simulink model "UAV_sync_known_sim"  (R2018b)
settings: Solver=ode23tb  StartTime=0.0  StopTime=35
values from neighbouring files (symbols this model uses):
  C_rho = 1.225    [SC42120_UAV_Preconditions.m]
  D0 = [M0 0 0 0 0 0 ... (first row only)    [SC42120_UAV_Preconditions.m]
  Derivative_gain_phi = 50    [SC42120_UAV_Preconditions.m]
  Derivative_gain_psi = 50    [SC42120_UAV_Preconditions.m]
  Derivative_gain_theta = 50    [SC42120_UAV_Preconditions.m]
  Derivative_gain_x = 50    [SC42120_UAV_Preconditions.m]
  Derivative_gain_y = 50    [SC42120_UAV_Preconditions.m]
  Derivative_gain_z = 50    [SC42120_UAV_Preconditions.m]
  G = 9.80665    [SC42120_UAV_Preconditions.m]
  g0 = [0;0;-M0*G;0;0;0]    [SC42120_UAV_Preconditions.m]
  I0 = [0.02 0 -0.01 ... (first row only)    [SC42120_UAV_Preconditions.m]
  I1 = [0.1 0 -0.01;0 0.05 0;-0.01 0 0.1]    [UAV_sync_known.m]    (also in UAV_sync_unknown.m; UAV_sync_unknown_Node1.m)
  InitWind = [0;0;0]    [SC42120_UAV_Preconditions.m]
  M0 = 10    [SC42120_UAV_Preconditions.m]
  M1 = 20    [UAV_sync_known.m]    (also in UAV_sync_unknown.m; UAV_sync_unknown_Node1.m)
  Proportional_phi = 50    [SC42120_UAV_Preconditions.m]
  Proportional_psi = 50    [SC42120_UAV_Preconditions.m]
  Proportional_theta = 50    [SC42120_UAV_Preconditions.m]
  Proportional_x = 50    [SC42120_UAV_Preconditions.m]
  Proportional_y = 50    [SC42120_UAV_Preconditions.m]
  Proportional_z = 50    [SC42120_UAV_Preconditions.m]
undefined symbols (not defined in the file or in its folder): Aero, APlane, Bxl, C, Ctr, deg, DiscIntNeverNeededParam, F, Guid, Init, Light, MIL, Path, rad, s, Trim, Utility
libraries: aerolibconvert2 x37, simulink x15, dspsigops x7, shared6dof x6, aerolibasang x4, simulink_extras x3, aerolibadyn x1, aerolibtransform2 x1, aerolibwind2 x1
(part 1 of 6)
settings Model: Creator=Muhammad Ridho Rosa  LastModifiedBy=Jesse
settings SolverCC: ZeroCrossAlgorithm=Adaptive
settings SFSimCC: SimUseLocalCustomCode=off
settings RTWCC: RTWUseLocalCustomCode=off
settings CodeAppCC: StateflowObjectComments=on

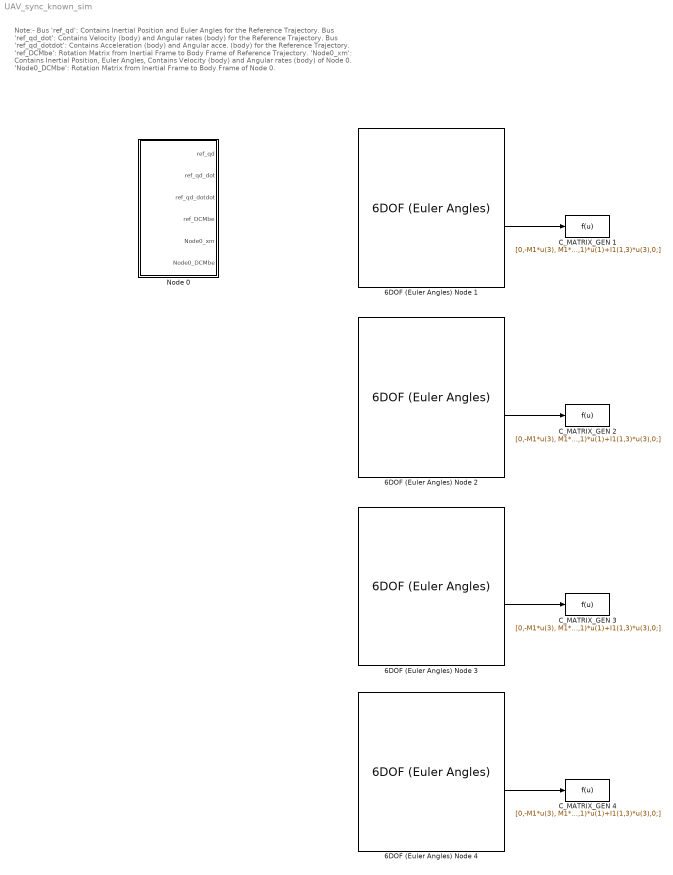
== system UAV_sync_known_sim ==
  note: Note:-
      | Bus 'ref_qd': Contains Inertial Position and Euler Angles for the Reference Trajectory.
      | Bus 'ref_qd_dot': Contains Velocity (body) and Angular rates (body) for the Reference Trajectory.
      | Bus 'ref_qd_dotdot': Contains Acceleration (body) and Angular acce. (body) for the Reference Trajectory.
      | 'ref_DCMbe': Rotation Matrix from Inertial Frame to Body Frame of Reference Trajectory.
      | 'Node0_xm': Contains Inertial Position, Euler Angles, Contains Velocity (body) and Angular rates (body) of Node 0.
      | 'Node0_DCMbe': Rotation Matrix from Inertial Frame to Body Frame of Node 0.
  6DOF (Euler Angles) Node 1 : shared6dof/6DOF (Euler Angles)  units=Metric (MKS)  mtype=Fixed  rep=Euler Angles  xme_0=init_pos1  Vm_0=init_vel1  eul_0=init_eul1  pm_0=init_ang1  mass_0=M1  mass_e=0.5  mass_f=2.0  inertia=I1  inertia_e=eye(3)  inertia_f=2*eye(3)  k_quat=1.0  vre_flag=on  abi_flag=on  aMode=0  xme_statename=''  Vm_statename=''  eul_statename=''  quat_statename=''  pm_statename=''  mass_statename=''
      settings: SourceProductBaseCode=AE
  6DOF (Euler Angles) Node 2 : shared6dof/6DOF (Euler Angles)  units=Metric (MKS)  mtype=Fixed  rep=Euler Angles  xme_0=init_pos2  Vm_0=init_vel2  eul_0=init_eul2  pm_0=init_ang2  mass_0=M2  mass_e=0.5  mass_f=2.0  inertia=I2  inertia_e=eye(3)  inertia_f=2*eye(3)  k_quat=1.0  vre_flag=on  abi_flag=on  aMode=0  xme_statename=''  Vm_statename=''  eul_statename=''  quat_statename=''  pm_statename=''  mass_statename=''
      settings: SourceProductBaseCode=AE
  6DOF (Euler Angles) Node 3 : shared6dof/6DOF (Euler Angles)  units=Metric (MKS)  mtype=Fixed  rep=Euler Angles  xme_0=init_pos3  Vm_0=init_vel3  eul_0=init_eul3  pm_0=init_ang3  mass_0=M3  mass_e=0.5  mass_f=2.0  inertia=I3  inertia_e=eye(3)  inertia_f=2*eye(3)  k_quat=1.0  vre_flag=on  abi_flag=on  aMode=0  xme_statename=''  Vm_statename=''  eul_statename=''  quat_statename=''  pm_statename=''  mass_statename=''
      settings: SourceProductBaseCode=AE
  6DOF (Euler Angles) Node 4 : shared6dof/6DOF (Euler Angles)  units=Metric (MKS)  mtype=Fixed  rep=Euler Angles  xme_0=init_pos4  Vm_0=init_vel4  eul_0=init_eul4  pm_0=init_ang4  mass_0=M4  mass_e=0.5  mass_f=2.0  inertia=I4  inertia_e=eye(3)  inertia_f=2*eye(3)  k_quat=1.0  vre_flag=on  abi_flag=on  aMode=0  xme_statename=''  Vm_statename=''  eul_statename=''  quat_statename=''  pm_statename=''  mass_statename=''
      settings: SourceProductBaseCode=AE
  C_MATRIX_GEN {1..4} (4 alike) : Fcn  Expr=[0,-M1*u(3), M1*u(2), 0,0,0; M1*u(3),0,-M1*u(1),0,0,0;-M1*u(2),M1*u(1),0,0,0,0;0,0,0,0,I1(3,3)*u(3)-I1(1,3)*u(1),-I1(2,2)*u(2);0,0,0,-I1(3,3)*u(3)+I1(1,3)*u(1),0,I1(1,1)*u(1)-I1(1,3)*u(3);0,0,0,I1(2,2)*u(2),-I1(1,1)*u(1)+I1(1,3)*u(3),0;]
  Node 0 : Subsystem
  wires:
  6DOF (Euler Angles) Node 1/6 -> C_MATRIX_GEN 1/1
  6DOF (Euler Angles) Node 2/6 -> C_MATRIX_GEN 2/1
  6DOF (Euler Angles) Node 3/6 -> C_MATRIX_GEN 3/1
  6DOF (Euler Angles) Node 4/6 -> C_MATRIX_GEN 4/1

== system UAV_sync_known_sim/Node 0 ==
  Bus Creator : BusCreator  Inputs=2
  Bus Creator1 : BusCreator  Inputs=2
  Bus Creator2 : BusCreator  Inputs=2
  Bus Creator3 : BusCreator  Inputs=4
  Bus Selector : BusSelector  OutputSignals=PlantData.Position (inertial),PlantData.Euler angles (rad),PlantData.Velocity (body),PlantData.Angular rates (body) (rad/s),PlantData.Accelerations (body/body),PlantData.Angular accelerations (body/body),PlantData.From inertial to body matrix
  Bus Selector1 : BusSelector  OutputSignals=Position (inertial),Euler angles (rad),Velocity (body),Angular rates (body),MatrixTransformation(Inertial-Body)
  Node 0 : Subsystem
  VF Approach : Subsystem
  ref_qd : Outport
  ref_qd_dot : Outport  Port=2
  ref_qd_dotdot : Outport  Port=3
  ref_DCMbe : Outport  Port=4
  Node0_xm : Outport  Port=5
  Node0_DCMbe : Outport  Port=6
  wires:
  VF Approach/1(VF_System_Parameters) -> Node 0/1(VF_System_Parameters)
  VF Approach/2(PlantData) -> Bus Selector/1
  Bus Selector/1 -> Bus Creator/1  "<Position (inertial)>"
  Bus Selector/2 -> Bus Creator/2  "<Euler angles (rad)>"
  Bus Creator/1 -> ref_qd/1
  Bus Selector/4 -> Bus Creator1/2  "<Angular rates (body) (rad/s)>"
  Bus Selector/3 -> Bus Creator1/1  "<Velocity (body)>"
  Bus Creator1/1 -> ref_qd_dot/1
  Bus Selector/6 -> Bus Creator2/2  "<Angular accelerations (body/body)>"
  Bus Selector/5 -> Bus Creator2/1  "<Accelerations (body/body)>"
  Bus Creator2/1 -> ref_qd_dotdot/1
  Bus Selector/7 -> ref_DCMbe/1  "<From inertial to body matrix>"
  Node 0/1(Node0_Data) -> Bus Selector1/1
  Bus Selector1/1 -> Bus Creator3/1  "<Position (inertial)>"
  Bus Selector1/3 -> Bus Creator3/3  "<Velocity (body)>"
  Bus Selector1/4 -> Bus Creator3/4  "<Angular rates (body)>"
  Bus Creator3/1 -> Node0_xm/1
  Bus Selector1/5 -> Node0_DCMbe/1  "<MatrixTransformation(Inertial-Body)>"
  Bus Selector1/2 -> Bus Creator3/2  "<Euler angles (rad)>"

== system UAV_sync_known_sim/Node 0/Node 0 ==
  note: Inverse Dynamics
  VF_System_Parameters : Inport
  6DOF (Euler Angles) : shared6dof/6DOF (Euler Angles)  units=Metric (MKS)  mtype=Fixed  rep=Euler Angles  xme_0=init_pos0  Vm_0=init_vel0  eul_0=init_eul0  pm_0=init_ang0  mass_0=M0  mass_e=0.5  mass_f=2.0  inertia=I0  inertia_e=eye(3)  inertia_f=2*eye(3)  k_quat=1.0  vre_flag=on  abi_flag=off  aMode=aMode  xme_statename=''  Vm_statename=''  eul_statename=''  quat_statename=''  pm_statename=''  mass_statename=''
      settings: SourceProductBaseCode=AE
  ALL_DATA2 : Goto  Commented=on  GotoTag=DERIVED_DATA
  Add : Sum
  Bus Creator : BusCreator  Inputs=10
  Constant8 : Constant  Value=M0*G
  Demux5 : Demux  Outputs=6
  Derived Data : Subsystem
  Gain : Gain  Gain=[1 1 -1]
  Inverse Dynamics Control : Subsystem
  Mux8 : Mux  Inputs=3
  Mux9 : Mux  Inputs=3
  Product : Product  Multiplication=Matrix(*)
  Subsystem : Subsystem
  Wind : Subsystem
  tau : Sum  Inputs=+++
  Node0_Data : Outport
  wires:
  Gain/1 -> Product/2, Bus Creator/3  "xyh"
  6DOF (Euler Angles)/1 -> Bus Creator/1  "Velocity (inertial)"
  Mux8/1 -> 6DOF (Euler Angles)/1
  6DOF (Euler Angles)/3 -> Bus Creator/4  "Euler angles (rad)"
  Bus Creator/1 -> [AIRCRAFT_DATA]
  6DOF (Euler Angles)/6 -> Bus Creator/7  "Angular rates (body)"
  6DOF (Euler Angles)/8 -> Bus Creator/9  "Acceleration (Body)"
  Mux9/1 -> 6DOF (Euler Angles)/2
  6DOF (Euler Angles)/7 -> Bus Creator/8  "Angular accelerations (body)"
  6DOF (Euler Angles)/5 -> Bus Creator/6  "Velocity (body)"
  6DOF (Euler Angles)/2 -> Gain/1, Bus Creator/2  "Position (inertial)"
  6DOF (Euler Angles)/4 -> Product/1, Bus Creator/5  "MatrixTransformation(Inertial-Body)"
  tau/1 -> Demux5/1
  Demux5/2 -> Mux8/2
  Demux5/4 -> Mux9/1
  Demux5/5 -> Mux9/2
  Demux5/6 -> Mux9/3
  [WIND_DATA] -> Derived Data/1(In1)
  [AIRCRAFT_DATA] -> Derived Data/2(In2)
  Derived Data/1(Derived_Condition) -> ALL_DATA2/1
  [AIRCRAFT_DATA] -> Wind/1(In1)
  Wind/1(Out1) -> [WIND_DATA]
  Inverse Dynamics Control/1(D_qddot) -> tau/1
  Inverse Dynamics Control/2(C_qdot) -> tau/2
  Inverse Dynamics Control/3(g(q)) -> tau/3
  Constant8/1 -> Add/2
  Demux5/3 -> Add/1
  Add/1 -> Mux8/3
  Demux5/1 -> Mux8/1
  [AIRCRAFT_DATA] -> Inverse Dynamics Control/2(Aircraft Data), Node0_Data/1
  VF_System_Parameters/1 -> Subsystem/1(VF_System_Parameters)
  Subsystem/1(References) -> Inverse Dynamics Control/1(References)
  Product/1 -> Bus Creator/10  "xyh_body"

== system UAV_sync_known_sim/Node 0/VF Approach ==
  note: Created by: Stefano Farì
      | Last edit: Mar 2018
  note: Fixed-wing UAV Simulator
  note: Ground Hit
  note: Wind
  note: To workspace
  note: MAIN
  AUTOPILOT : Subsystem
  BIXLER DYNAMICS : Subsystem
  Bus Selector3 : BusSelector  OutputSignals=PlantData.xyh_body,PlantData.Euler angles (rad),PlantData.Velocity (body),PlantData.Angular rates (body) (rad/s),PlantData.Accelerations (body/body),PlantData.Angular accelerations (body/body)
  ENVIRONMENT : Subsystem
  GROUND HIT : Subsystem
  MANUAL INPUTS : Subsystem
  Mux : Mux  Inputs=6
  PATH FOLLOWING : Subsystem
  PATH MANAGER : Subsystem
  TO WORKSPACE : Subsystem
  VF_System_Parameters : Outport
  PlantData : Outport  Port=2
  wires:
  MANUAL INPUTS/2(EnvData.) -> BIXLER DYNAMICS/2(EnvData)
  [PlantData] -> PATH MANAGER/1(PlantData)
  MANUAL INPUTS/4(VF.) -> BIXLER DYNAMICS/4(VF)
  [VF] -> TO WORKSPACE/4(VF)
  MANUAL INPUTS/3(GuidData.) -> BIXLER DYNAMICS/3(GuidData)
  [EnvData] -> PATH MANAGER/3(EnvData)
  [PlantData] -> PlantData/1, Bus Selector3/1
  BIXLER DYNAMICS/4(GuidData.) -> [GuidData]
  MANUAL INPUTS/1(CtrBus.) -> BIXLER DYNAMICS/1(ControlActions)
  AUTOPILOT/3(VF.) -> MANUAL INPUTS/3(VF)
  PATH MANAGER/2(DerCond.) -> PATH FOLLOWING/2(DerCond)
  PATH FOLLOWING/1("PlantData. ") -> AUTOPILOT/1(PlantData)
  AUTOPILOT/4(GuidData.) -> MANUAL INPUTS/4(GuidData)
  [GuidData] -> TO WORKSPACE/5(GuidData)
  [DerCond] -> TO WORKSPACE/2(DerCond)
  PATH FOLLOWING/5(GuidData.) -> AUTOPILOT/5(GuidData)
  BIXLER DYNAMICS/5(VF.) -> [VF]
  PATH FOLLOWING/2("DerCond. ") -> AUTOPILOT/2(DerCond)
  BIXLER DYNAMICS/1(PlantData.) -> [PlantData]
  [PlantData] -> GROUND HIT/1(PlantData)
  [PlantData] -> ENVIRONMENT/1(PlantData)
  BIXLER DYNAMICS/3(ControlBus.) -> [ControlBus]
  AUTOPILOT/2(EnvData.) -> MANUAL INPUTS/2(EnvData)
  PATH MANAGER/1(Plantdata.) -> PATH FOLLOWING/1(PlantData)
  PATH MANAGER/4(GuidData.) -> PATH FOLLOWING/4(GuidData)
  ENVIRONMENT/1(EnvData) -> [EnvData]
  PATH FOLLOWING/4(VF.) -> AUTOPILOT/4(VF)
  Bus Selector3/4 -> Mux/4  "<Angular rates (body) (rad/s)>"
  PATH MANAGER/3(EnvData.) -> PATH FOLLOWING/3(EnvData)
  [PlantData] -> TO WORKSPACE/1(PlantData)
  [DerCond] -> PATH MANAGER/2(DerCond)
  BIXLER DYNAMICS/2(DerCond.) -> [DerCond]
  [EnvData] -> TO WORKSPACE/6(EnvData)
  [ControlBus] -> TO WORKSPACE/3(ControlBus)
  AUTOPILOT/1(CtrBus.) -> MANUAL INPUTS/1(CtrBus)
  PATH FOLLOWING/3(EnvData.) -> AUTOPILOT/3(EnvData)
  Mux/1 -> VF_System_Parameters/1
  Bus Selector3/1 -> Mux/1  "<xyh_body>"
  Bus Selector3/2 -> Mux/2  "<Euler angles (rad)>"
  Bus Selector3/3 -> Mux/3  "<Velocity (body)>"
  Bus Selector3/5 -> Mux/5  "<Accelerations (body/body)>"
  Bus Selector3/6 -> Mux/6  "<Angular accelerations (body/body)>"

== system UAV_sync_known_sim/Node 0/Node 0/Derived Data ==
  note: WAE = Wind Angle Error
  In1 : Inport
  In2 : Inport  Port=2
  Bus Creator2 : BusCreator  Inputs=7
  Bus Selector : BusSelector  OutputSignals=WindVelocity(Body)
  Bus Selector5 : BusSelector  OutputSignals=Velocity (body),Velocity (inertial),Euler angles (rad)
  Constant9 : Constant  Value=C_rho
  Dynamic Pressure : aerolibasang/Dynamic Pressure
  "Incidence, Sideslip, & Airspeed" : aerolibasang/Incidence, Sideslip, & Airspeed
      settings: SourceProductName=Aerospace Blockset
  Scope : Scope
  Selector : Selector  InputPortWidth=3  IndexOptions=Index vector (dialog)  Indices=3  OutputSizes=1
  Selector1 : Selector  InputPortWidth=3  IndexOptions=Index vector (dialog)  Indices=2  OutputSizes=1
  Selector3 : Selector  InputPortWidth=3  IndexOptions=Index vector (dialog)  Indices=1  OutputSizes=1
  Sum2 : Sum  Inputs=|-+
  Sum4 : Sum  Inputs=+-|
  Sum5 : Sum  Inputs=+-|
  Trigonometric Function1 : Trigonometry  Operator=atan2
  Derived_Condition : Outport
  wires:
  In2/1 -> Bus Selector5/1
  "Incidence, Sideslip, & Airspeed"/2 -> Sum5/2, Bus Creator2/2  "beta"
  "Incidence, Sideslip, & Airspeed"/1 -> Bus Creator2/1  "alpha"
  Dynamic Pressure/1 -> Bus Creator2/4  "qbar"
  Sum2/1 -> "Incidence, Sideslip, & Airspeed"/1
  Constant9/1 -> Dynamic Pressure/2
  Bus Selector5/2 -> Selector1/1, Selector3/1  "<Velocity (inertial)>"
  Trigonometric Function1/1 -> Sum4/1, Bus Creator2/5  "course_angle"
  Bus Selector5/3 -> Selector/1  "<Euler angles (rad)>"
  Selector/1 -> Sum4/2
  Sum5/1 -> Bus Creator2/7  "WAE"
  "Incidence, Sideslip, & Airspeed"/3 -> Scope/1, Bus Creator2/3  "Va"
  Sum4/1 -> Sum5/1, Bus Creator2/6  "crab_angle"
  Bus Selector5/1 -> Dynamic Pressure/1, Sum2/2  "<Velocity (body)>"
  Bus Creator2/1 -> Derived_Condition/1
  In1/1 -> Bus Selector/1
  Bus Selector/1 -> Sum2/1  "<WindVelocity(Body)>"
  Selector1/1 -> Trigonometric Function1/1
  Selector3/1 -> Trigonometric Function1/2

== system UAV_sync_known_sim/Node 0/Node 0/Inverse Dynamics Control ==
  References : Inport
  Aircraft Data : Inport  Port=2
  Constant8 : Constant  Value=g0
  Inverse Dynamic 1 : Subsystem
  Inverse Dynamic 2 : Subsystem
  D_qddot : Outport
  C_qdot : Outport  Port=2
  g(q) : Outport  Port=3
  wires:
  Inverse Dynamic 1/1(D_qddot) -> D_qddot/1
  References/1 -> Inverse Dynamic 1/1(References)
  Aircraft Data/1 -> Inverse Dynamic 2/1(Aricraft Data), Inverse Dynamic 1/2(Aircraft Data)
  Inverse Dynamic 2/1(C_qdot) -> C_qdot/1
  Constant8/1 -> g(q)/1

== system UAV_sync_known_sim/Node 0/Node 0/Subsystem ==
  VF_System_Parameters : Inport
  Bus Creator1 : BusCreator  Inputs=18
  Demux : Demux  Outputs=18
  References : Outport
  wires:
  VF_System_Parameters/1 -> Demux/1
  Demux/7 -> Bus Creator1/7  "xdot_ref_final"
  Demux/6 -> Bus Creator1/6  "psi_ref_final"
  Demux/9 -> Bus Creator1/9  "hdot_ref_final"
  Demux/18 -> Bus Creator1/18  "psiddot_ref_final"
  Bus Creator1/1 -> References/1
  Demux/1 -> Bus Creator1/1  "x_ref _final"
  Demux/4 -> Bus Creator1/4  "phi_ref_final"
  Demux/5 -> Bus Creator1/5  "theta_ref_final"
  Demux/2 -> Bus Creator1/2  "y_ref_final"
  Demux/3 -> Bus Creator1/3  "h_ref_final"
  Demux/8 -> Bus Creator1/8  "ydot_ref_final"
  Demux/14 -> Bus Creator1/14  "yddot_ref_final"
  Demux/16 -> Bus Creator1/16  "phiddot_ref_final"
  Demux/15 -> Bus Creator1/15  "hddot_ref_final"
  Demux/10 -> Bus Creator1/10  "phidot_ref_final"
  Demux/13 -> Bus Creator1/13  "xddot_ref_final"
  Demux/17 -> Bus Creator1/17  "thetaddot_ref_final"
  Demux/12 -> Bus Creator1/12  "psidot_ref_final"
  Demux/11 -> Bus Creator1/11  "thetadot_ref_final"

== system UAV_sync_known_sim/Node 0/Node 0/Wind ==
  In1 : Inport
  Bus Creator1 : BusCreator  Inputs=1
  Bus Selector4 : BusSelector  OutputSignals=MatrixTransformation(Inertial-Body)
  Constant1 : Constant  Value=InitWind
  Product : Product  Multiplication=Matrix(*)
  Out1 : Outport
  wires:
  Constant1/1 -> Product/2
  In1/1 -> Bus Selector4/1
  Bus Selector4/1 -> Product/1  "<MatrixTransformation(Inertial-Body)>"
  Product/1 -> Bus Creator1/1  "WindVelocity(Body)"
  Bus Creator1/1 -> Out1/1

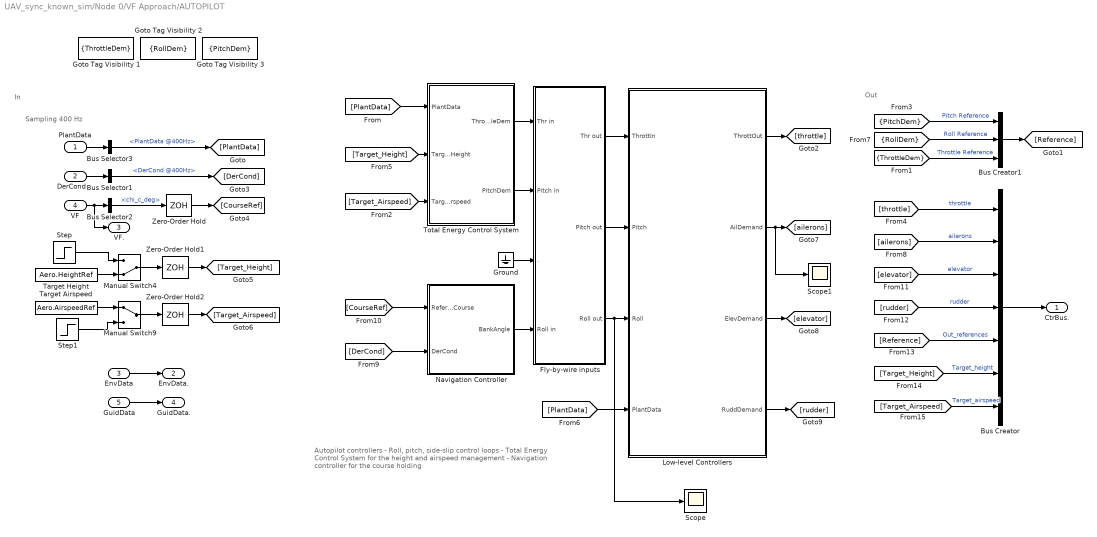
== system UAV_sync_known_sim/Node 0/VF Approach/AUTOPILOT ==
  note: In
  note: Out
  note: Autopilot controllers
      |
      | - Roll, pitch, side-slip control loops
      | - Total Energy Control System for the height and airspeed management
      | - Navigation controller for the course holding
  note: Sampling 400 Hz
  PlantData : Inport
  DerCond : Inport  Port=2
  EnvData : Inport  Port=3
  VF : Inport  Port=4
  GuidData : Inport  Port=5
  Bus Creator : BusCreator  Inputs=7
  Bus Creator1 : BusCreator  Inputs=3
  Bus Selector1 : BusSelector  OutputSignals=DerCond @400Hz
  Bus Selector2 : BusSelector  OutputSignals=chi_c_deg
  Bus Selector3 : BusSelector  OutputSignals=PlantData @400Hz
  Fly-by-wire inputs : Subsystem
  Goto Tag Visibility 1 : GotoTagVisibility  GotoTag=ThrottleDem
  Goto Tag Visibility 2 : GotoTagVisibility  GotoTag=RollDem
  Goto Tag Visibility 3 : GotoTagVisibility  GotoTag=PitchDem
  Ground : Ground
  Low-level Controllers : Subsystem
  Manual Switch4 : ManualSwitch  CurrentSetting=0
  Manual Switch9 : ManualSwitch
  Navigation Controller : Subsystem
  Scope : Scope
  Scope1 : Scope
  Step : Step  Time=10  Before=50  After=80  SampleTime=0
  Step1 : Step  Time=10  Before=15  After=20  SampleTime=0
  Target Airspeed : Constant  Value=Aero.AirspeedRef
  Target Height : Constant  Value=Aero.HeightRef
  Total Energy Control System : Subsystem
  Zero-Order Hold : ZeroOrderHold  SampleTime=1/400
  Zero-Order Hold1 : ZeroOrderHold  SampleTime=1/400
  Zero-Order Hold2 : ZeroOrderHold  SampleTime=1/400
  CtrBus. : Outport
  EnvData. : Outport  Port=2
  VF. : Outport  Port=3
  GuidData. : Outport  Port=4
  wires:
  Bus Creator1/1 -> [Reference]
  PlantData/1 -> Bus Selector3/1
  Low-level Controllers/4(RuddDemand) -> [rudder]
  Low-level Controllers/3(ElevDemand) -> [elevator]
  Low-level Controllers/2(AilDemand) -> Scope1/1, [ailerons]
  Low-level Controllers/1(ThrottOut) -> [throttle]
  [RollDem] -> Bus Creator1/2  "Roll Reference"
  [CourseRef] -> Navigation Controller/1(ReferenceCourse)
  [PlantData] -> Low-level Controllers/4(PlantData)
  Bus Selector1/1 -> [DerCond]  "<DerCond @400Hz>"
  DerCond/1 -> Bus Selector1/1
  [DerCond] -> Navigation Controller/2(DerCond)
  Bus Selector3/1 -> [PlantData]  "<PlantData @400Hz>"
  Manual Switch4/1 -> Zero-Order Hold1/1
  Manual Switch9/1 -> Zero-Order Hold2/1
  Step/1 -> Manual Switch4/1
  Target Height/1 -> Manual Switch4/2
  Target Airspeed/1 -> Manual Switch9/1
  Step1/1 -> Manual Switch9/2
  [PitchDem] -> Bus Creator1/1  "Pitch Reference"
  Zero-Order Hold/1 -> [CourseRef]
  [PlantData] -> Total Energy Control System/1(PlantData)
  EnvData/1 -> EnvData./1
  GuidData/1 -> GuidData./1
  VF/1 -> VF./1, Bus Selector2/1
  Bus Selector2/1 -> Zero-Order Hold/1  "<chi_c_deg>"
  [ThrottleDem] -> Bus Creator1/3  "Throttle Reference"
  Zero-Order Hold1/1 -> [Target_Height]
  Zero-Order Hold2/1 -> [Target_Airspeed]
  Total Energy Control System/1(ThrottleDem) -> Fly-by-wire inputs/1(Thr in)
  Total Energy Control System/2(PitchDem) -> Fly-by-wire inputs/2(Pitch in)
  Navigation Controller/1(BankAngle) -> Fly-by-wire inputs/4(Roll in)
  Fly-by-wire inputs/1(Thr out) -> Low-level Controllers/1(ThrottIn)
  Fly-by-wire inputs/2(Pitch out) -> Low-level Controllers/2(Pitch)
  Ground/1 -> Fly-by-wire inputs/3(.)
  [Target_Height] -> Total Energy Control System/2(Target_Height)
  [Target_Airspeed] -> Total Energy Control System/3(Target_Airspeed)
  [ailerons] -> Bus Creator/2  "ailerons"
  [throttle] -> Bus Creator/1  "throttle"
  [elevator] -> Bus Creator/3  "elevator"
  [rudder] -> Bus Creator/4  "rudder"
  [Reference] -> Bus Creator/5  "Out_references"
  [Target_Height] -> Bus Creator/6  "Target_height"
  [Target_Airspeed] -> Bus Creator/7  "Target_airspeed"
  Bus Creator/1 -> CtrBus./1
  Fly-by-wire inputs/3(Roll out) -> Low-level Controllers/3(Roll), Scope/1

== system UAV_sync_known_sim/Node 0/VF Approach/BIXLER DYNAMICS ==
  note: This sub-block contains the dynamics of the aircraft.
      |
      | - All the states and quantities of interest are contained in the Bus signal PlantData.
      | - The derived conditions such as Airspeed, Angle of Attack, and Side-slip angle, are contained in Bus signal DerCond .
      | - The Bus EnvData contains the wind quantities of interest.
      | - The dynamical model is continuous, but the Buses are sampled to feed the discrete-time control system.
      | - The parameters of this block are contained in parameters/parameters_aero.
  ControlActions : Inport
  EnvData : Inport  Port=2
  GuidData : Inport  Port=3
  VF : Inport  Port=4
  Actuator Dynamics : Subsystem
  Bus Creator1 : BusCreator  Inputs='qbar','alpha','beta','Va','Course','CrabAngle','WAE'
  Bus Selector : BusSelector  OutputSignals=throttle
  Derived Conditions : Subsystem
  RUBBISH BIN : Subsystem
  Sampling : Subsystem
  "Sampling " : Subsystem
  Throttle Dynamics : Subsystem
  Vehicle Airframe : Subsystem
  PlantData. : Outport
  DerCond. : Outport  Port=2
  ControlBus. : Outport  Port=3
  GuidData. : Outport  Port=4
  VF. : Outport  Port=5
  wires:
  Bus Creator1/1 -> "Sampling "/1(Cont.), [DerCond]  "DerCond"
  Bus Selector/1 -> Throttle Dynamics/1(In)  "<throttle>"
  Throttle Dynamics/1(Out) -> Vehicle Airframe/1(Throttle_cmd)  "throttle"
  ControlActions/1 -> ControlBus./1, Bus Selector/1, Actuator Dynamics/1(In)
  Actuator Dynamics/1(Out) -> Vehicle Airframe/2(ControlActions)
  Vehicle Airframe/1(PlantData) -> [PlantData], Sampling/1(Cont.)  "PlantData"
  Sampling/1(Cont.+Disc.) -> PlantData./1
  "Sampling "/1(Cont.+Disc.) -> DerCond./1
  GuidData/1 -> GuidData./1
  VF/1 -> VF./1
  [PlantData] -> Derived Conditions/2(PlantData)
  EnvData/1 -> Derived Conditions/1(EnvData)
  Derived Conditions/1(qbar) -> Bus Creator1/1  "qbar"
  Derived Conditions/2(alpha) -> Bus Creator1/2  "alpha"
  Derived Conditions/4(Va) -> Bus Creator1/4  "Va"
  Derived Conditions/3(beta) -> Bus Creator1/3  "beta"
  Derived Conditions/5(CourseAngle) -> Bus Creator1/5  "Course"
  Derived Conditions/6(CrabAngle) -> Bus Creator1/6  "CrabAngle"
  Derived Conditions/7(WAE) -> Bus Creator1/7  "WAE"
  [DerCond] -> Vehicle Airframe/3(DerCond)

== system UAV_sync_known_sim/Node 0/VF Approach/ENVIRONMENT ==
  note: Wind slowly time varying
  note: Dynamic wind
  note: Constant wind
  PlantData : Inport
  Bus Creator : BusCreator  Inputs=4
  Bus Selector1 : BusSelector  OutputSignals=xyh,Velocity (inertial),From inertial to body matrix
  Bus Selector2 : BusSelector  OutputSignals=From inertial to body matrix
  Bus Selector3 : BusSelector  OutputSignals=PlantData
  Bus Selector4 : BusSelector  OutputSignals=From inertial to body matrix
  Constant1 : Constant  Value=Init.windConst
  Dot Product : DotProduct  InputSameDT=on  OutDataTypeStr=Inherit: Inherit via internal rule
  Dryden Wind Turbulence Model (Continuous (+q +r)) : aerolibwind2/Dryden Wind Turbulence Model  (Continuous (+q -r))  units=Metric (MKS)  spec=MIL-F-8785C  model=Continuous Dryden (+q +r)  W20=10  Wdeg=135  TurbProb=10^-2 - Light  L_high=533.4  Wingspan=Bxl.b  ts=0.1  Seed=[23341 23342 23343 23344]  T_on=on
      settings: SourceProductName=Aerospace Blockset
  Height : Selector  InputPortWidth=3  IndexOptions=Index vector (dialog)  Indices=3  OutputSizes=1
  Init.DryOnOff : Gain  Gain=Init.DryOnOff
  "Init.DryOnOff " : Gain  Gain=Init.DryOnOff
  Init.WTimevar : Gain  Gain=Init.WTimevar
  Product : Product  Multiplication=Matrix(*)
  "Product " : Product  Multiplication=Matrix(*)
  Slowly time varying wind gen. : Subsystem
  Sum1 : Sum  Inputs=|++
  Sum3 : Sum  Inputs=|++
  Vt : Sqrt  SaturateOnIntegerOverflow=on
  EnvData : Outport
  wires:
  Bus Selector1/1 -> Height/1  "<xyh>"
  Bus Selector1/2 -> Dot Product/2, Dot Product/1  "<Velocity (inertial)>"
  Bus Selector1/3 -> Dryden Wind Turbulence Model (Continuous (+q +r))/3  "<From inertial to body matrix>"
  Bus Selector3/1 -> Bus Selector4/1, Bus Selector1/1, Bus Selector2/1  "<PlantData>"
  Height/1 -> Dryden Wind Turbulence Model (Continuous (+q +r))/1  "Altitude"
  Dot Product/1 -> Vt/1
  Vt/1 -> Dryden Wind Turbulence Model (Continuous (+q +r))/2  "Speed"
  Sum1/1 -> Bus Creator/3, Sum3/2  "Wind velocity (dyn) (body)"
  Constant1/1 -> Product/2
  Bus Creator/1 -> EnvData/1
  "Init.DryOnOff "/1 -> Bus Creator/4  "Wind ang rate (dyn) (body)"
  Sum3/1 -> Bus Creator/2  "Wind total (body)"
  Dryden Wind Turbulence Model (Continuous (+q +r))/1 -> Init.DryOnOff/1
  Bus Selector2/1 -> Product/1  "<From inertial to body matrix>"
  Dryden Wind Turbulence Model (Continuous (+q +r))/2 -> "Init.DryOnOff "/1
  PlantData/1 -> Bus Selector3/1
  Product/1 -> Bus Creator/1, Sum3/1  "Wind velocity (sta) (body)"
  Bus Selector4/1 -> "Product "/1  "<From inertial to body matrix>"
  Init.WTimevar/1 -> Sum1/2  "Wind slowly time varying"
  Init.DryOnOff/1 -> Sum1/1
  "Product "/1 -> Init.WTimevar/1
  Slowly time varying wind gen./1(Out1) -> "Product "/2

== system UAV_sync_known_sim/Node 0/VF Approach/GROUND HIT ==
  PlantData : Inport
  Bus Selector1 : BusSelector  OutputSignals=xyh
  Bus Selector3 : BusSelector  OutputSignals=PlantData
  Constant : Constant  Value=0
  Relational Operator : RelationalOperator  Operator=<=  OutDataTypeStr=boolean  RndMeth=Simplest
  Selector : Selector  InputPortWidth=3  IndexOptions=Index vector (dialog)  Indices=3  OutputSizes=1
  Stop Simulation : Stop
  wires:
  PlantData/1 -> Bus Selector3/1
  Selector/1 -> Relational Operator/1
  Bus Selector1/1 -> Selector/1  "<xyh>"
  Constant/1 -> Relational Operator/2
  Relational Operator/1 -> Stop Simulation/1
  Bus Selector3/1 -> Bus Selector1/1  "<PlantData>"

== system UAV_sync_known_sim/Node 0/VF Approach/MANUAL INPUTS ==
  note: Manual control
      |
      | The switches below enable (up position) or disable (down position) the manual control in the Visual Interface sub-block.
      | (default: down)
  note: Open-loop inputs
      |
      | The switches below enables a custom input from the Workspace (timeseries data type) to the control surfaces.
  note: Trim condition
      |
      | The sub-block below allows to try the actuators configuration for a trimmed flight.
  CtrBus : Inport
  EnvData : Inport  Port=2
  VF : Inport  Port=3
  GuidData : Inport  Port=4
  Bus Creator : BusCreator  Inputs=7
  Bus Selector : BusSelector  OutputSignals=throttle,ailerons,elevator,rudder
  Bus Selector1 : BusSelector  OutputSignals=Out_references,Target_height,Target_airspeed
  "CtrBus " : InportShadow
  From Workspace1 : FromWorkspace  Commented=on  VariableName=LogData.RCIN.ElevDem_IN  SampleTime=0.001
  From Workspace2 : FromWorkspace  Commented=on  VariableName=LogData.RCIN.RuddDem_IN  SampleTime=0.001
  From Workspace3 : FromWorkspace  Commented=on  VariableName=LogData.RCIN.ThrottleDem_IN  SampleTime=0.001
  From Workspace4 : FromWorkspace  Commented=on  VariableName=LogData.RCIN.AilDem_IN  SampleTime=0.001
  Goto4 : Goto  Commented=on  GotoTag=throttle
  Manual Switch{,1..7} (8 alike) : ManualSwitch  CurrentSetting=0
  Manual_cmd{,4..6} (4 alike) : Constant  Value=0
  Trim conditions : Subsystem
  CtrBus. : Outport
  EnvData. : Outport  Port=2
  GuidData. : Outport  Port=3
  VF. : Outport  Port=4
  wires:
  Manual Switch4/1 -> Goto4/1, Bus Creator/1  "throttle"
  Manual Switch7/1 -> Bus Creator/3  "elevator"
  Manual_cmd/1 -> Manual Switch/1
  Manual_cmd4/1 -> Manual Switch1/1
  Manual Switch5/1 -> Bus Creator/2  "ailerons"
  Manual Switch6/1 -> Bus Creator/4  "rudder"
  Manual_cmd6/1 -> Manual Switch3/1
  Manual_cmd5/1 -> Manual Switch2/1
  Bus Creator/1 -> CtrBus./1
  Manual Switch1/1 -> Manual Switch5/2  "ailerons"
  Manual Switch2/1 -> Manual Switch7/2  "elevator"
  Manual Switch3/1 -> Manual Switch6/2  "rudder"
  From Workspace3/1 -> Manual Switch4/1
  Manual Switch/1 -> Manual Switch4/2
  Bus Selector/1 -> Trim conditions/1(throttle)  "<throttle>"
  Trim conditions/1(throttout) -> Manual Switch/2
  Bus Selector/2 -> Trim conditions/2(ail)  "<ailerons>"
  Bus Selector/3 -> Trim conditions/3(elev)  "<elevator>"
  Bus Selector/4 -> Trim conditions/4(rudd)  "<rudder>"
  Trim conditions/4(ruddout) -> Manual Switch3/2
  Trim conditions/2(ailout) -> Manual Switch1/2
  Trim conditions/3(elevout) -> Manual Switch2/2
  EnvData/1 -> EnvData./1
  From Workspace4/1 -> Manual Switch5/1
  From Workspace1/1 -> Manual Switch7/1
  From Workspace2/1 -> Manual Switch6/1
  GuidData/1 -> GuidData./1
  VF/1 -> VF./1
  CtrBus/1 -> Bus Selector/1
  "CtrBus "/1 -> Bus Selector1/1
  Bus Selector1/1 -> Bus Creator/5  "<Out_references>"
  Bus Selector1/2 -> Bus Creator/6  "<Target_height>"
  Bus Selector1/3 -> Bus Creator/7  "<Target_airspeed>"

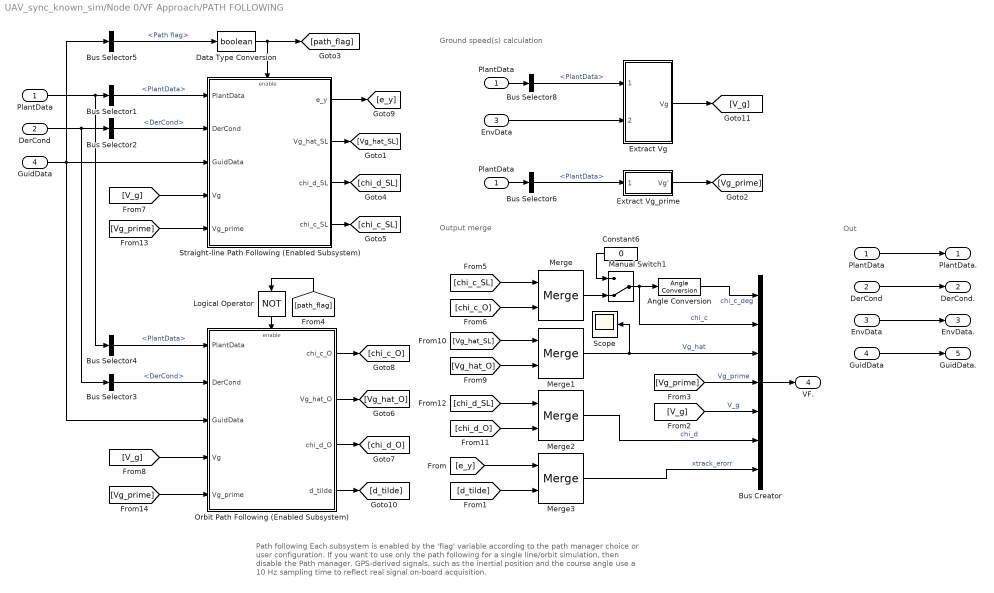
== system UAV_sync_known_sim/Node 0/VF Approach/PATH FOLLOWING ==
  note: Out
  note: Ground speed(s) calculation
  note: Output merge
  note: Path following
      |
      | Each subsystem is enabled by the 'flag' variable according to the path manager choice or user configuration.
      | If you want to use only the path following for a single line/orbit simulation, then disable the Path manager.
      |
      | GPS-derived signals, such as the inertial position and the course angle use a 10 Hz sampling time to reflect real signal on-board acquisition.
  PlantData : Inport
  DerCond : Inport  Port=2
  EnvData : Inport  Port=3
  GuidData : Inport  Port=4
  Angle Conversion : aerolibconvert2/Angle Conversion  IU=rad  OU=deg
  Bus Creator : BusCreator  Inputs=7
  Bus Selector{1,4,6,8} (4 alike) : BusSelector  OutputSignals=PlantData
  Bus Selector2 : BusSelector  OutputSignals=DerCond
  Bus Selector3 : BusSelector  OutputSignals=DerCond
  Bus Selector5 : BusSelector  OutputSignals=Path flag
  Constant6 : Constant  Value=0
  Data Type Conversion : DataTypeConversion  OutDataTypeStr=boolean
  "DerCond " : InportShadow  Port=2
  "EnvData " : InportShadow  Port=3
  Extract Vg : Subsystem
  Extract Vg_prime : Subsystem
  "GuidData " : InportShadow  Port=4
  Logical Operator : Logic  Operator=NOT  AllPortsSameDT=off  OutDataTypeStr=boolean
  Manual Switch1 : ManualSwitch  CurrentSetting=0
  Merge{,1..3} (4 alike) : Merge
  Orbit Path Following (Enabled Subsystem) : Subsystem  TreatAsAtomicUnit=on
  "PlantData " : InportShadow
  "PlantData  " : InportShadow
  "PlantData   " : InportShadow
  Scope : Scope
  Straight-line Path Following (Enabled Subsystem) : Subsystem  TreatAsAtomicUnit=on
  "PlantData. " : Outport
  "DerCond. " : Outport  Port=2
  EnvData. : Outport  Port=3
  VF. : Outport  Port=4
  GuidData. : Outport  Port=5
  wires:
  Merge/1 -> Manual Switch1/2
  Constant6/1 -> Manual Switch1/1
  EnvData/1 -> EnvData./1
  PlantData/1 -> Bus Selector4/1, Bus Selector1/1
  Bus Selector1/1 -> Straight-line Path Following (Enabled Subsystem)/1(PlantData)  "<PlantData>"
  DerCond/1 -> Bus Selector2/1, Bus Selector3/1
  Bus Creator/1 -> VF./1
  Manual Switch1/1 -> Bus Creator/2, Angle Conversion/1  "chi_c"
  Logical Operator/1 -> Orbit Path Following (Enabled Subsystem)/Enable
  Bus Selector4/1 -> Orbit Path Following (Enabled Subsystem)/1(PlantData)  "<PlantData>"
  Bus Selector3/1 -> Orbit Path Following (Enabled Subsystem)/2(DerCond)  "<DerCond>"
  Data Type Conversion/1 -> [path_flag], Straight-line Path Following (Enabled Subsystem)/Enable
  [path_flag] -> Logical Operator/1
  Bus Selector2/1 -> Straight-line Path Following (Enabled Subsystem)/2(DerCond)  "<DerCond>"
  Merge1/1 -> Bus Creator/3, Scope/1  "Vg_hat"
  [Vg_prime] -> Bus Creator/4  "Vg_prime"
  Straight-line Path Following (Enabled Subsystem)/2(Vg_hat_SL) -> [Vg_hat_SL]
  Straight-line Path Following (Enabled Subsystem)/3(chi_d_SL) -> [chi_d_SL]
  Straight-line Path Following (Enabled Subsystem)/4(chi_c_SL) -> [chi_c_SL]
  Orbit Path Following (Enabled Subsystem)/2(Vg_hat_O) -> [Vg_hat_O]
  Orbit Path Following (Enabled Subsystem)/3(chi_d_O) -> [chi_d_O]
  Orbit Path Following (Enabled Subsystem)/1(chi_c_O) -> [chi_c_O]
  [chi_c_SL] -> Merge/1
  [chi_c_O] -> Merge/2
  [Vg_hat_O] -> Merge1/2
  [Vg_hat_SL] -> Merge1/1
  [chi_d_O] -> Merge2/2
  [chi_d_SL] -> Merge2/1
  Merge2/1 -> Bus Creator/6  "chi_d"
  Angle Conversion/1 -> Bus Creator/1  "chi_c_deg"
  Straight-line Path Following (Enabled Subsystem)/1(e_y) -> [e_y]
  [e_y] -> Merge3/1
  Orbit Path Following (Enabled Subsystem)/4(d_tilde) -> [d_tilde]
  [d_tilde] -> Merge3/2
  Merge3/1 -> Bus Creator/7  "xtrack_erorr"
  GuidData/1 -> Bus Selector5/1, Orbit Path Following (Enabled Subsystem)/3(GuidData), Straight-line Path Following (Enabled Subsystem)/3(GuidData)
  Bus Selector5/1 -> Data Type Conversion/1  "<Path flag>"
  "DerCond "/1 -> "DerCond. "/1
  "GuidData "/1 -> GuidData./1
  "PlantData "/1 -> "PlantData. "/1
  Extract Vg_prime/1(Vg') -> [Vg_prime]
  Bus Selector6/1 -> Extract Vg_prime/1(PlantData)  "<PlantData>"
  [V_g] -> Bus Creator/5  "V_g"
  Extract Vg/1(Vg) -> [V_g]
  "PlantData  "/1 -> Bus Selector6/1
  [V_g] -> Straight-line Path Following (Enabled Subsystem)/4(Vg)
  [V_g] -> Orbit Path Following (Enabled Subsystem)/4(Vg)
  [Vg_prime] -> Straight-line Path Following (Enabled Subsystem)/5(Vg_prime)
  [Vg_prime] -> Orbit Path Following (Enabled Subsystem)/5(Vg_prime)
  "EnvData "/1 -> Extract Vg/2(EnvData)
  "PlantData   "/1 -> Bus Selector8/1
  Bus Selector8/1 -> Extract Vg/1(PlantData)  "<PlantData>"

== system UAV_sync_known_sim/Node 0/VF Approach/PATH MANAGER ==
  note: Path following only
  note: Path manager
  PlantData : Inport
  DerCond : Inport  Port=2
  EnvData : Inport  Port=3
  Bus Selector : BusSelector  OutputSignals=PlantData.Position (inertial)
  Constant : Constant  Value=Path.onOff
  Constant1 : Constant  Value=Path.onOff
  Data Type Conversion : DataTypeConversion  OutDataTypeStr=boolean
  Enabled Subsystem : Subsystem  TreatAsAtomicUnit=on
  Fcn : Fcn  Commented=on  Expr=u(1)
  Fcn1 : Fcn  Commented=on  Expr=u(2)
  Logical Operator : Logic  Operator=NOT  AllPortsSameDT=off  OutDataTypeStr=boolean
  Merge : Merge
  Path Following data : Subsystem  TreatAsAtomicUnit=on
  XY Graph : simulink/Sinks/XY Graph  Commented=on  xmin=-50  xmax=600  ymin=-50  ymax=600  st=0.1
  Plantdata. : Outport
  DerCond. : Outport  Port=2
  EnvData. : Outport  Port=3
  GuidData. : Outport  Port=4
  wires:
  PlantData/1 -> Bus Selector/1, Plantdata./1
  DerCond/1 -> DerCond./1
  EnvData/1 -> EnvData./1
  Bus Selector/1 -> Fcn1/1, Fcn/1, Enabled Subsystem/1(xy)  "<Position (inertial)>"
  Merge/1 -> GuidData./1
  Constant/1 -> Data Type Conversion/1
  Data Type Conversion/1 -> Enabled Subsystem/Enable
  Constant1/1 -> Logical Operator/1
  Logical Operator/1 -> Path Following data/Enable
  Enabled Subsystem/1(GuidData) -> Merge/1
  Path Following data/1(GuidData) -> Merge/2
  Fcn/1 -> XY Graph/1
  Fcn1/1 -> XY Graph/2

== system UAV_sync_known_sim/Node 0/VF Approach/TO WORKSPACE ==
  PlantData : Inport
  DerCond : Inport  Port=2
  ControlBus : Inport  Port=3
  VF : Inport  Port=4
  GuidData : Inport  Port=5
  EnvData : Inport  Port=6
  Bus Creator : BusCreator  Inputs=6
  Bus Selector4 : BusSelector  OutputSignals=DerCond
  Bus Selector5 : BusSelector  OutputSignals=PlantData
  Sample at 0.01s : ZeroOrderHold  SampleTime=0.01
  To Workspace2 : ToWorkspace  VariableName=SimOut  SaveFormat=Timeseries  SampleTime=-1
      settings: Save2DSignal=2-D array (concatenate along first dimension)
  wires:
  Bus Creator/1 -> Sample at 0.01s/1
  Bus Selector5/1 -> Bus Creator/1  "<PlantData>"
  PlantData/1 -> Bus Selector5/1
  ControlBus/1 -> Bus Creator/3  "ControlBus"
  DerCond/1 -> Bus Selector4/1
  Bus Selector4/1 -> Bus Creator/2  "<DerCond>"
  GuidData/1 -> Bus Creator/5  "GuidData"
  VF/1 -> Bus Creator/4  "VF"
  EnvData/1 -> Bus Creator/6  "EnvData"
  Sample at 0.01s/1 -> To Workspace2/1

== system UAV_sync_known_sim/Node 0/Node 0/Inverse Dynamics Control/Inverse Dynamic 1 ==
  References : Inport
  Aircraft Data : Inport  Port=2
  Add2 : Sum  Inputs=-+
  Bus Selector2 : BusSelector  OutputSignals=xyh_body,Euler angles (rad),Velocity (body),Angular rates (body)
  Bus Selector3 : BusSelector  OutputSignals=xddot_ref_final,yddot_ref_final,hddot_ref_final,phiddot_ref_final,thetaddot_ref_final,psiddot_ref_final
  Constant10 : Constant  Value=D0
  Gain3 : Gain  Gain=-1
  Inner Controller : Subsystem
  Mux1 : Mux  Inputs=6
  Mux5 : Mux  Inputs=6
  Product1 : Product  Multiplication=Matrix(*)
  Subsystem : Subsystem
  D_qddot : Outport
  wires:
  Aircraft Data/1 -> Bus Selector2/1
  Subsystem/4(e_phi) -> Inner Controller/4(e_phi)
  Subsystem/3(e_z) -> Inner Controller/3(e_z)
  Subsystem/5(e_theta) -> Inner Controller/5(e_theta)
  Bus Selector2/1 -> Subsystem/1(<xyh>)  "<xyh_body>"
  Subsystem/2(e_y) -> Inner Controller/2(e_y)
  Mux5/1 -> Add2/1
  Subsystem/6(e_psi) -> Inner Controller/6(e_psi)
  Product1/1 -> D_qddot/1
  Add2/1 -> Product1/2
  Inner Controller/3(act3) -> Gain3/1
  Constant10/1 -> Product1/1
  Mux1/1 -> Add2/2
  Bus Selector2/2 -> Subsystem/2(<Euler angles (rad)>)  "<Euler angles (rad)>"
  Inner Controller/1(act1) -> Mux5/1
  Subsystem/1(e_x) -> Inner Controller/1(e_x)
  Inner Controller/5(act5) -> Mux5/5
  Inner Controller/6(act6) -> Mux5/6
  Inner Controller/4(act4) -> Mux5/4
  Bus Selector2/3 -> Subsystem/3(velocity)  "<Velocity (body)>"
  Subsystem/7(e_xdot) -> Inner Controller/7(e_xdot)
  Bus Selector2/4 -> Subsystem/4(angular_rate)  "<Angular rates (body)>"
  Subsystem/8(e_zdot) -> Inner Controller/8(e_zdot)
  Subsystem/9(e_phidot) -> Inner Controller/9(e_phidot)
  Subsystem/10(e_thetadot) -> Inner Controller/10(e_thetadot)
  Subsystem/11(e_psidot) -> Inner Controller/11(e_psidot)
  Subsystem/12(e_ydot) -> Inner Controller/12(e_ydot)
  Inner Controller/2(act2) -> Mux5/2
  Bus Selector3/1 -> Mux1/1  "<xddot_ref_final>"
  Bus Selector3/2 -> Mux1/2  "<yddot_ref_final>"
  Bus Selector3/3 -> Mux1/3  "<hddot_ref_final>"
  Bus Selector3/4 -> Mux1/4  "<phiddot_ref_final>"
  Bus Selector3/5 -> Mux1/5  "<thetaddot_ref_final>"
  Bus Selector3/6 -> Mux1/6  "<psiddot_ref_final>"
  References/1 -> Subsystem/5(Reference), Bus Selector3/1
  Gain3/1 -> Mux5/3

== system UAV_sync_known_sim/Node 0/Node 0/Inverse Dynamics Control/Inverse Dynamic 2 ==
  Aricraft Data : Inport
  Bus Selector1 : BusSelector  OutputSignals=Velocity (body),Angular rates (body)
  Constant1 : Constant  Value=I0(3)
  Constant2 : Constant  Value=I0(1)
  Constant3 : Constant  Value=M0
  Constant4 : Constant  Value=I0(5)
  Constant5 : Constant  Value=I0(9)
  Constant6 : Constant  Value=[0 0 0;0 0 0;0 0 0]
  Constant7 : Constant  Value=0
  Matrix Concatenate : Concatenate  Mode=Multidimensional array  ConcatenateDimension=2
  Matrix Concatenate1 : Concatenate  Mode=Multidimensional array  ConcatenateDimension=2
  Matrix Concatenate2 : Concatenate  Mode=Multidimensional array
  Mux1 : Mux  Inputs=2
  Product2 : Product  Multiplication=Matrix(*)
  Rot_Matrix [3x3] : Subsystem
  Trans_Matrix [3x3] : Subsystem
  p : Fcn  Expr=u(1)
  q : Fcn  Expr=u(2)
  r : Fcn  Expr=u(3)
  C_qdot : Outport
  wires:
  Aricraft Data/1 -> Bus Selector1/1
  Matrix Concatenate/1 -> Matrix Concatenate2/1
  Matrix Concatenate1/1 -> Matrix Concatenate2/2
  Rot_Matrix [3x3]/1(Out1) -> Matrix Concatenate1/2
  Constant7/1 -> Trans_Matrix [3x3]/4(zero), Rot_Matrix [3x3]/4(Zero)
  Constant3/1 -> Trans_Matrix [3x3]/5(M)
  r/1 -> Rot_Matrix [3x3]/3(r), Trans_Matrix [3x3]/3(r)
  Constant2/1 -> Rot_Matrix [3x3]/5(I1)
  Trans_Matrix [3x3]/1(Out1) -> Matrix Concatenate/1
  Bus Selector1/1 -> Mux1/1  "<Velocity (body)>"
  Constant4/1 -> Rot_Matrix [3x3]/6(I5)
  Matrix Concatenate2/1 -> Product2/1
  Bus Selector1/2 -> Mux1/2, p/1, q/1, r/1  "<Angular rates (body)>"
  Constant5/1 -> Rot_Matrix [3x3]/7(I9)
  Constant6/1 -> Matrix Concatenate/2, Matrix Concatenate1/1
  q/1 -> Rot_Matrix [3x3]/2(q), Trans_Matrix [3x3]/2(q)
  p/1 -> Rot_Matrix [3x3]/1(p), Trans_Matrix [3x3]/1(p)
  Product2/1 -> C_qdot/1
  Mux1/1 -> Product2/2
  Constant1/1 -> Rot_Matrix [3x3]/8(I3_I7)

== system UAV_sync_known_sim/Node 0/VF Approach/AUTOPILOT/Fly-by-wire inputs ==
  note: Put here your custom inputs
  Thr in : Inport
  Pitch in : Inport  Port=2
  . : Inport  Port=3
  Roll in : Inport  Port=4
  Constant : Constant  Commented=on  Value=0
  Dummy port : Terminator
  From Workspace : FromWorkspace  Commented=on  VariableName=LogData.RCIN.Throttle_IN  SampleTime=0.001
  From Workspace1 : FromWorkspace  Commented=on  VariableName=LogData.RCIN.Pitch_IN  SampleTime=0.001
  From Workspace2 : FromWorkspace  Commented=on  VariableName=LogData.RCIN.Roll_IN  SampleTime=0.001
  Manual Switch1 : ManualSwitch  CurrentSetting=0
  Manual Switch2 : ManualSwitch
  Manual Switch3 : ManualSwitch
  Manual Switch4 : ManualSwitch
  Thr out : Outport
  Pitch out : Outport  Port=2
  Roll out : Outport  Port=3
  tag scope: PitchDem=scoped, RollDem=scoped, ThrottleDem=scoped
  wires:
  Manual Switch3/1 -> Pitch out/1
  Manual Switch1/1 -> Thr out/1
  Pitch in/1 -> [PitchDem], Manual Switch3/1
  From Workspace/1 -> Manual Switch1/1
  Manual Switch2/1 -> [RollDem], Roll out/1
  Roll in/1 -> Manual Switch2/1
  From Workspace1/1 -> Manual Switch3/2
  Thr in/1 -> [ThrottleDem], Manual Switch1/2
  Constant/1 -> Manual Switch4/2
  From Workspace2/1 -> Manual Switch4/1
  Manual Switch4/1 -> Manual Switch2/2
  ./1 -> Dummy port/1

== system UAV_sync_known_sim/Node 0/VF Approach/AUTOPILOT/Low-level Controllers ==
  ThrottIn : Inport  Unit=%
  Pitch : Inport  Port=2  Unit=deg
  Roll : Inport  Port=3  Unit=deg
  PlantData : Inport  Port=4
  Angle Conversion1 : aerolibconvert2/Angle Conversion  IU=rad  OU=deg
  Angle Conversion2 : aerolibconvert2/Angle Conversion  IU=rad  OU=deg
  Angular Velocity Conversion : aerolibconvert2/Angular Velocity Conversion  IU=rad/s  OU=deg/s
      settings: SourceProductName=Aerospace Blockset
  Angular Velocity Conversion1 : aerolibconvert2/Angular Velocity Conversion  IU=rad/s  OU=deg/s
      settings: SourceProductName=Aerospace Blockset
  Bus Selector : BusSelector  OutputSignals=Euler angles (rad)
  Bus Selector1 : BusSelector  OutputSignals=Angular rates (body) (rad/s)
  Bus Selector2 : BusSelector  OutputSignals=Euler angles (rad)
  Bus Selector3 : BusSelector  OutputSignals=Angular rates (body) (rad/s)
  Bus Selector5 : BusSelector  OutputSignals=Angular rates (body) (rad/s)
  Bus Selector6 : BusSelector  OutputSignals=Euler angles (rad)
  Bus Selector7 : BusSelector  OutputSignals=Accelerations (body/body)
  Get scaling factor : Subsystem
  Pitch controller : Subsystem
  Roll controller : Subsystem
  Side-slip angle controller : Subsystem
  ThrottOut : Outport  Unit=%
  AilDemand : Outport  Port=2  Unit=deg
  ElevDemand : Outport  Port=3  Unit=deg
  RuddDemand : Outport  Port=4  Unit=deg
  wires:
  Bus Selector/1 -> Angle Conversion1/1  "<Euler angles (rad)>"
  Roll controller/1(AilDemand) -> [AilDem], AilDemand/1
  Bus Selector1/1 -> Angular Velocity Conversion1/1  "<Angular rates (body) (rad/s)>"
  Bus Selector2/1 -> Angle Conversion2/1  "<Euler angles (rad)>"
  Bus Selector3/1 -> Angular Velocity Conversion/1  "<Angular rates (body) (rad/s)>"
  Pitch controller/1(ElevDemand) -> ElevDemand/1
  Get scaling factor/1(Scaler) -> Roll controller/4(Scaler), Side-slip angle controller/4(Scaler), Pitch controller/4(Scaler)
  Bus Selector7/1 -> Side-slip angle controller/3(accel_y)  "<Accelerations (body/body)>"
  Bus Selector6/1 -> Side-slip angle controller/2("Euler angles ")  "<Euler angles (rad)>"
  Bus Selector5/1 -> Side-slip angle controller/1(Yaw_rate)  "<Angular rates (body) (rad/s)>"
  [PlantData] -> Bus Selector1/1, Bus Selector2/1, Bus Selector3/1, Bus Selector5/1, Bus Selector6/1, Bus Selector7/1, Bus Selector/1
  Pitch/1 -> [PitchRef]
  PlantData/1 -> [PlantData]
  ThrottIn/1 -> ThrottOut/1
  Angle Conversion2/1 -> Pitch controller/2(EulerAngles)
  Angular Velocity Conversion/1 -> Pitch controller/3(AngularRates)
  Angle Conversion1/1 -> Roll controller/2(Euler angles)
  Angular Velocity Conversion1/1 -> Roll controller/3(AngularRates)
  Roll/1 -> [RollRef]
  [PitchRef] -> Pitch controller/1(PitchReference)
  [RollRef] -> Roll controller/1(RollReference)
  [AilDem] -> Side-slip angle controller/5(AilDemand)
  Side-slip angle controller/1(RudderDemand) -> RuddDemand/1

== system UAV_sync_known_sim/Node 0/VF Approach/AUTOPILOT/Navigation Controller ==
  note: Activate bias only if you have troubles with undesired settling orbits.
  ReferenceCourse : Inport  Unit=deg
  DerCond : Inport  Port=2
  Angle Conversion : aerolibconvert2/Angle Conversion  IU=rad  OU=deg
  Bias : Bias  Bias=360
  Bus Selector : BusSelector  OutputSignals=Course
  Constant : Constant  Value=45
  Discrete PID Controller : simulink/Continuous/PID Controller  Controller=PD  TimeDomain=Discrete-time  SampleTime=Ctr.TS  IntegratorMethod=Forward Euler  FilterMethod=Forward Euler  Form=Parallel  UseFilter=on  ControllerParametersSource=internal  P=Ctr.Hdg2Roll.NAV_ROLL_P  I=0.01  D=Ctr.Hdg2Roll.NAV_ROLL_D  N=2*pi*20  InitialConditionSource=internal  InitialConditionForIntegrator=0  InitialConditionForFilter=0  ExternalReset=none  LimitOutput=on  UpperSaturationLimit=45  LowerSaturationLimit=-45  LinearizeAsGain=off  AntiWindupMode=clamping  Kb=1  TrackingMode=off  Kt=1  PParamMin=[]  PParamMax=[]  IParamMin=[]  IParamMax=[]  DParamMin=[]  DParamMax=[]  NParamMin=[]  NParamMax=[]  KbParamMin=[]  KbParamMax=[]  KtParamMin=[]  KtParamMax=[]  POutMin=[]  POutMax=[]  IOutMin=[]  IOutMax=[]  DOutMin=[]  DOutMax=[]  NOutMin=[]  NOutMax=[]  KbOutMin=[]  KbOutMax=[]  KtOutMin=[]  KtOutMax=[]  IntegratorOutMin=[]  IntegratorOutMax=[]  FilterOutMin=[]  FilterOutMax=[]  SumOutMin=[]  SumOutMax=[]  SumI1OutMin=[]  SumI1OutMax=[]  SumI2OutMin=[]  SumI2OutMax=[]  SumI3OutMin=[]  SumI3OutMax=[]  SumDOutMin=[]  SumDOutMax=[]  SaturationOutMin=[]  SaturationOutMax=[]  IntegratorContinuousStateAttributes=''  IntegratorStateMustResolveToSignalObject=off  IntegratorRTWStateStorageClass=Auto  FilterContinuousStateAttributes=''  FilterStateMustResolveToSignalObject=off  FilterRTWStateStorageClass=Auto  DifferentiatorICPrevScaledInput=0  DifferentiatorOutMin=[]  DifferentiatorOutMax=[]
  Manual Switch : ManualSwitch  CurrentSetting=0
  Manual Switch1 : ManualSwitch
  PID : Subsystem  Commented=on
  Scope : Scope
  Scope1 : Scope
  Scope2 : Scope  NumInputPorts=2
  Step : Step  Time=10  After=90  SampleTime=0
  Sum : Sum  Inputs=|+-
  Unwrap : Subsystem
  Unwrap1 : dspsigops/Unwrap  tol=pi  InputProcessing=Columns as channels (frame based)  running=off
  Zero-Order Hold : ZeroOrderHold  SampleTime=1/400
  BankAngle : Outport  Unit=deg
  wires:
  Bus Selector/1 -> Unwrap1/1  "<Course>"
  Discrete PID Controller/1 -> Manual Switch1/1, Scope/1
  DerCond/1 -> Bus Selector/1
  Unwrap1/1 -> Angle Conversion/1  "chi_measured"
  Sum/1 -> Scope1/1, Discrete PID Controller/1
  Angle Conversion/1 -> Sum/2, Scope2/2
  ReferenceCourse/1 -> Manual Switch/2
  Unwrap/1(Out) -> Scope2/1, Sum/1
  Manual Switch/1 -> Bias/1
  Step/1 -> Zero-Order Hold/1
  Zero-Order Hold/1 -> Manual Switch/1
  Manual Switch1/1 -> BankAngle/1
  Constant/1 -> Manual Switch1/2
  Bias/1 -> Unwrap/1(In)
